simulink model "simul1_challenge"  (R2022b)
settings: Solver=FixedStepAuto  StartTime=0.0  StopTime=20  FixedStep=0.001  RelTol=1e-3
undefined symbols (not defined in the file): awu, degs2rpm, der, end_step, National_Instruments, PCI, pid, sens, simul, Ts
libraries: sldrtlib x3
settings Model: SimulationMode=external  ExtModeTrigDuration=50001  ExtModeTrigDurationFloating=50001  Creator=perondavid  LastModifiedBy=david
settings DataIOCC: LoggingToFile=on
settings HardwareCC: ProdBitPerLong=64  ProdHWDeviceType=Intel->x86-64 (Linux 64)
settings RTWCC: Description=Simulink Desktop Real-Time  SystemTargetFile=sldrt.tlc  TemplateMakefile=sldrt.tmf  RTWCompilerOptimization=on
settings CodeAppCC: MaxIdLength=95
settings SimulinkDesktopRealTimeCC: TargetLibSuffix=_sldrt.a  TargetPreCompLibLocation=C:\Program Files\MATLAB\R2022b\toolbox\sldrt\lib\win64

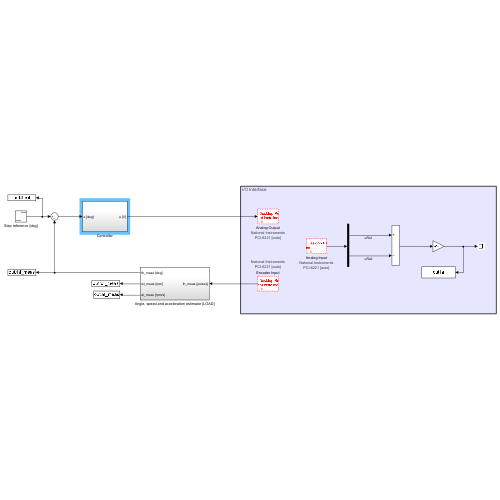
[thumbnail: Simulink's stored preview of the top-level diagram]
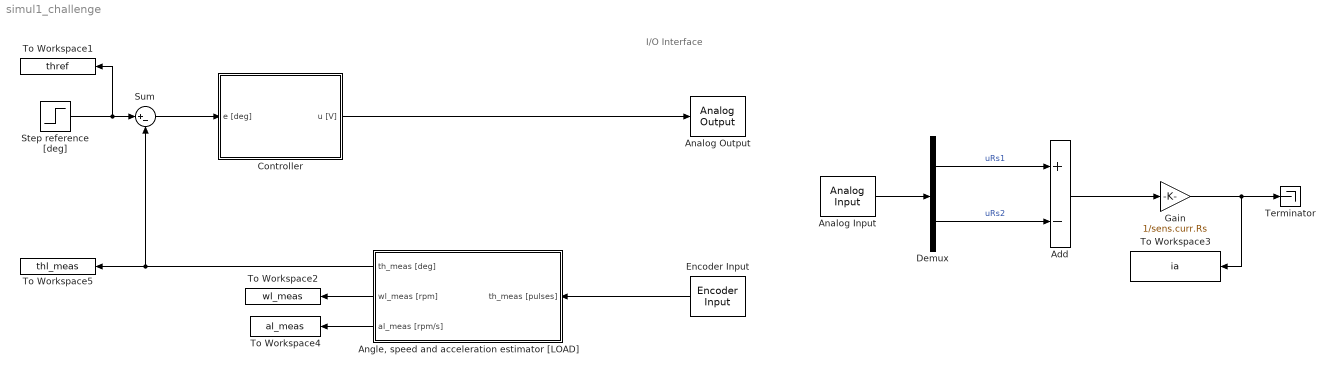
== system simul1_challenge ==
  note: I/O Interface
  Add : Sum  Inputs=+-
  Analog Input : sldrtlib/Analog Input  SampleTime=-1  MaxMissedTicks=10  ShowMissedTicks=off  YieldWhenWaiting=off  DrvName=National_Instruments/PCI-6221  DrvAddress=4294967295  DrvOptions=[0 0 0 2 0]  Channels=[1, 2]  RangeMode=1  VoltRange=1  DataType=1
      settings: AttributesFormatString=National Instruments\nPCI-6221 [auto]
  Analog Output : sldrtlib/Analog Output  SampleTime=-1  MaxMissedTicks=10  ShowMissedTicks=off  YieldWhenWaiting=off  DrvName=National_Instruments/PCI-6221  DrvAddress=4294967295  DrvOptions=[0 0 0 2 0]  Channels=1  RangeMode=1  VoltRange=1  InitialValue=0  FinalValue=0
      settings: AttributesFormatString=National Instruments\nPCI-6221 [auto]
  "Angle, speed and acceleration estimator [LOAD]" : Subsystem
  Controller : Subsystem
  Demux : Demux  Outputs=2
  Encoder Input : sldrtlib/Encoder Input  SampleTime=-1  MaxMissedTicks=10  ShowMissedTicks=off  YieldWhenWaiting=off  DrvName=National_Instruments/PCI-6221  DrvAddress=4294967295  DrvOptions=[0 0 0 2 0]  Channels=1  QuadMode=3  IndexPulse=1  InputFilter=Inf  DataType=1
      settings: AttributesFormatString=National Instruments\nPCI-6221 [auto]
  Gain : Gain  Gain=1/sens.curr.Rs
  Step reference [deg] : Step  After=simul.stepdeg
  Sum : Sum  Inputs=|+-
  Terminator : Terminator
  To Workspace1 : ToWorkspace  VariableName=thref  SaveFormat=Structure With Time  SampleTime=Ts
  To Workspace2 : ToWorkspace  VariableName=wl_meas  SaveFormat=Structure With Time  SampleTime=Ts
  To Workspace3 : ToWorkspace  VariableName=ia  SaveFormat=Structure With Time  SampleTime=Ts
  To Workspace4 : ToWorkspace  VariableName=al_meas  SaveFormat=Structure With Time  SampleTime=Ts
  To Workspace5 : ToWorkspace  VariableName=thl_meas  SaveFormat=Structure With Time  SampleTime=Ts
  wires:
  Demux/1 -> Add/1  "uRs1"
  Demux/2 -> Add/2  "uRs2"
  Add/1 -> Gain/1
  Gain/1 -> To Workspace3/1, Terminator/1
  Analog Input/1 -> Demux/1
  Sum/1 -> Controller/1(e [deg])
  Controller/1(u [V]) -> Analog Output/1
  Step reference [deg]/1 -> To Workspace1/1, Sum/1
  "Angle, speed and acceleration estimator [LOAD]"/3(al_meas [rpm/s]) -> To Workspace4/1
  "Angle, speed and acceleration estimator [LOAD]"/2(wl_meas [rpm]) -> To Workspace2/1
  "Angle, speed and acceleration estimator [LOAD]"/1(th_meas [deg]) -> To Workspace5/1, Sum/2
  Encoder Input/1 -> "Angle, speed and acceleration estimator [LOAD]"/1(th_meas [pulses])

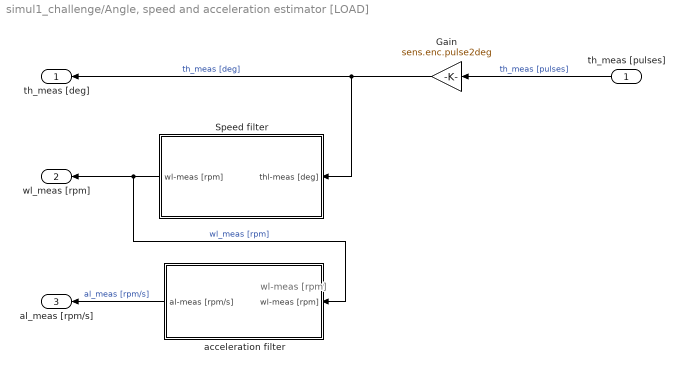
== system simul1_challenge/Angle, speed and acceleration estimator [LOAD] ==
  note: wl-meas [rpm]
  th_meas [pulses] : Inport
  Gain : Gain  Gain=sens.enc.pulse2deg
  Speed filter : Subsystem
  acceleration filter : Subsystem
  th_meas [deg] : Outport
  wl_meas [rpm] : Outport  Port=2
  al_meas [rpm/s] : Outport  Port=3
  wires:
  Speed filter/1(wl-meas [rpm]) -> acceleration filter/1(wl-meas [rpm]), wl_meas [rpm]/1  "wl_meas [rpm]"
  th_meas [pulses]/1 -> Gain/1  "th_meas [pulses]"
  Gain/1 -> Speed filter/1(thl-meas [deg]), th_meas [deg]/1  "th_meas [deg]"
  acceleration filter/1(al-meas [rpm/s]) -> al_meas [rpm/s]/1  "al_meas [rpm/s]"

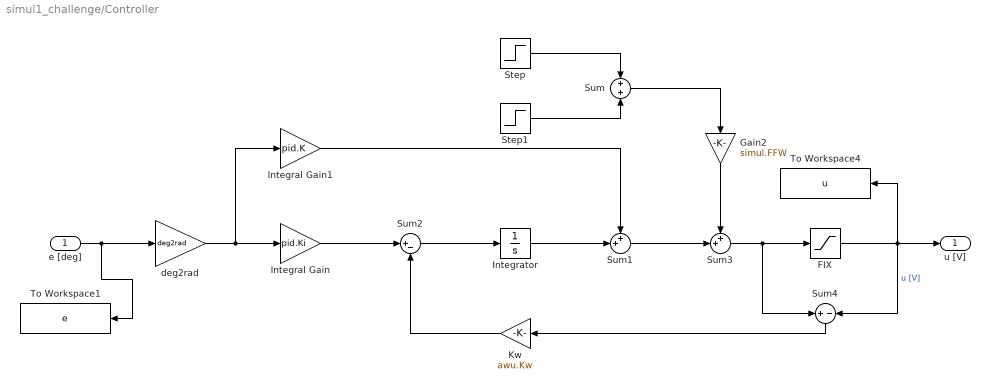
== system simul1_challenge/Controller ==
  e [deg] : Inport
  "FIX " : Saturate  UpperLimit=10  LowerLimit=-10
  Gain2 : Gain  Gain=simul.FFW
  Integral Gain : Gain  Gain=pid.Ki
  Integral Gain1 : Gain  Gain=pid.K
  Integrator : Integrator
  Kw : Gain  Gain=awu.Kw
  Step : Step  After=10  SampleTime=Ts
  Step1 : Step  Time=end_step  After=-10  SampleTime=Ts
  Sum : Sum
  Sum1 : Sum  Inputs=++|
  Sum2 : Sum  Inputs=|+-
  Sum3 : Sum  Inputs=++|
  Sum4 : Sum  Inputs=+-
  To Workspace1 : ToWorkspace  VariableName=e  SaveFormat=Structure With Time  SampleTime=Ts
  To Workspace4 : ToWorkspace  VariableName=u  SaveFormat=Structure With Time  SampleTime=Ts
  deg2rad : Gain  Gain=deg2rad
  u [V] : Outport
  wires:
  deg2rad/1 -> Integral Gain1/1, Integral Gain/1
  e [deg]/1 -> To Workspace1/1, deg2rad/1
  Gain2/1 -> Sum3/1
  Integrator/1 -> Sum1/2
  Step/1 -> Sum/1
  Step1/1 -> Sum/2
  Sum/1 -> Gain2/1
  Sum1/1 -> Sum3/2
  Integral Gain1/1 -> Sum1/1
  Sum3/1 -> Sum4/1, "FIX "/1
  "FIX "/1 -> Sum4/2, To Workspace4/1, u [V]/1  "u [V]"
  Integral Gain/1 -> Sum2/1
  Kw/1 -> Sum2/2
  Sum4/1 -> Kw/1
  Sum2/1 -> Integrator/1

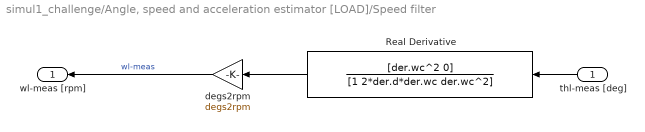
== system simul1_challenge/Angle, speed and acceleration estimator [LOAD]/Speed filter ==
  thl-meas [deg] : Inport
  Real Derivative : TransferFcn  Numerator=[der.wc^2 0]  Denominator=[1 2*der.d*der.wc der.wc^2]
  degs2rpm : Gain  Gain=degs2rpm
  wl-meas [rpm] : Outport
  wires:
  thl-meas [deg]/1 -> Real Derivative/1
  degs2rpm/1 -> wl-meas [rpm]/1  "wl-meas"
  Real Derivative/1 -> degs2rpm/1

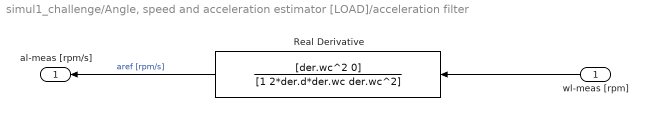
== system simul1_challenge/Angle, speed and acceleration estimator [LOAD]/acceleration filter ==
  wl-meas [rpm] : Inport
  Real Derivative : TransferFcn  Numerator=[der.wc^2 0]  Denominator=[1 2*der.d*der.wc der.wc^2]
  al-meas [rpm/s] : Outport
  wires:
  wl-meas [rpm]/1 -> Real Derivative/1
  Real Derivative/1 -> al-meas [rpm/s]/1  "aref [rpm/s]"
